simulink library "LIBRARY_SAD"  (R2025b)
settings: Solver=VariableStepAuto  StartTime=0.0  StopTime=10.0  RelTol=1e-3
values from neighbouring files (symbols this model uses):
  c = astroConstants(5)*1e3    [SCRIPT_SAD_DEMO.m]
  eps_E = deg2rad(astroConstants(63))    [SCRIPT_SAD_DEMO.m]
  F0 = 237    [SCRIPT_SAD_DEMO.m]
  F_e = 1358    [SCRIPT_SAD_DEMO.m]
  g = zeros(N, N+1)    [SCRIPT_SAD_DEMO.m]
  h = zeros(N, N+1)    [SCRIPT_SAD_DEMO.m]
  j_B = [0.01; 0.05; 0.01]    [SCRIPT_SAD_DEMO.m]
  JD0 = juliandate(startTime)    [SCRIPT_SAD_DEMO.m]
  mu = astroConstants(13)    [SCRIPT_SAD_DEMO.m]
  n = sqrt( (mu/ (a)^3))    [SCRIPT_SAD_DEMO.m]
  N = 13    [SCRIPT_SAD_DEMO.m]
  n_sun = 2*pi/T_sun    (= 1.99238499086e-07)    [SCRIPT_SAD_DEMO.m]
  r_sun = 1*AU    [SCRIPT_SAD_DEMO.m]
  Re = astroConstants(23)    [SCRIPT_SAD_DEMO.m]
  SRP = SRP_nom    [SCRIPT_SAD_DEMO.m]
  t0 = 0    [SCRIPT_SAD_DEMO.m]
  theta = 0    [SCRIPT_SAD_DEMO.m]
  w0 = w0_nom    [SCRIPT_SAD_DEMO.m]
  w_E = deg2rad(15.04)/3600    [SCRIPT_SAD_DEMO.m]
undefined symbols (not defined in the file or in its folder): g0_1, g1_1, h1_1, Ix, Iy, Iz, phi0, psi0, theta0
libraries: matrix_library x13, lIBRARY_SAD_SAD x12, $bdroot x5, LIBRARY_SAD_SAD x3, simulink x1
(part 2 of 2)

== system LIBRARY_SAD/Solar Radiation Torque (SRP)/Panel 3 ==
  Constant : Constant  Value=SRP.panel3.A
  Constant1 : Constant  Value=SRP.panel3.N_hat
  Constant2 : Constant  Value=SRP.panel3.rho_s
  Constant3 : Constant  Value=SRP.panel3.rho_d
  A_i : Outport
  N_B_hat_i : Outport  Port=2
  rho_s_i : Outport  Port=3
  rho_d_i : Outport  Port=4
  wires:
  Constant/1 -> A_i/1
  Constant1/1 -> N_B_hat_i/1
  Constant2/1 -> rho_s_i/1
  Constant3/1 -> rho_d_i/1

== system LIBRARY_SAD/Solar Radiation Torque (SRP)/Panel 4 ==
  Constant : Constant  Value=SRP.panel4.A
  Constant1 : Constant  Value=SRP.panel4.N_hat
  Constant2 : Constant  Value=SRP.panel4.rho_s
  Constant3 : Constant  Value=SRP.panel4.rho_d
  A_i : Outport
  N_B_hat_i : Outport  Port=2
  rho_s_i : Outport  Port=3
  rho_d_i : Outport  Port=4
  wires:
  Constant3/1 -> rho_d_i/1
  Constant2/1 -> rho_s_i/1
  Constant1/1 -> N_B_hat_i/1
  Constant/1 -> A_i/1

== system LIBRARY_SAD/Two-body Dynamics (keplerian elements)/Conic Equation ==
  a : Inport
  e : Inport  Port=2
  theta : Inport  Port=3
  Constant : Constant  Value=2
  Constant1 : Constant
  Constant2 : Constant
  Cos : Trigonometry  Operator=cos
  Divide : Product  Inputs=*/
  Power : Math  Operator=pow
  Product : Product
  Product1 : Product
  Sum : Sum  Inputs=+-
  Sum1 : Sum  Inputs=+-
  r : Outport
  wires:
  a/1 -> Product/1
  e/1 -> Product1/1, Power/1
  Constant/1 -> Power/2
  Power/1 -> Sum/2
  Constant1/1 -> Sum/1
  Sum/1 -> Product/2
  Product/1 -> Divide/1
  Divide/1 -> r/1
  Constant2/1 -> Sum1/1
  theta/1 -> Cos/1
  Cos/1 -> Product1/2
  Product1/1 -> Sum1/2
  Sum1/1 -> Divide/2

== system LIBRARY_SAD/Two-body Dynamics (keplerian elements)/Orbital Period ==
  a : Inport
  mu : Inport  Port=2
  Constant : Constant  Value=3
  Divide : Product  Inputs=*/
  Gain : Gain  Gain=2*pi
  Power : Math  Operator=pow
  Sqrt : Sqrt
  T : Outport
  wires:
  a/1 -> Power/1
  Constant/1 -> Power/2
  Power/1 -> Divide/1
  mu/1 -> Divide/2
  Divide/1 -> Sqrt/1
  Sqrt/1 -> Gain/1
  Gain/1 -> T/1

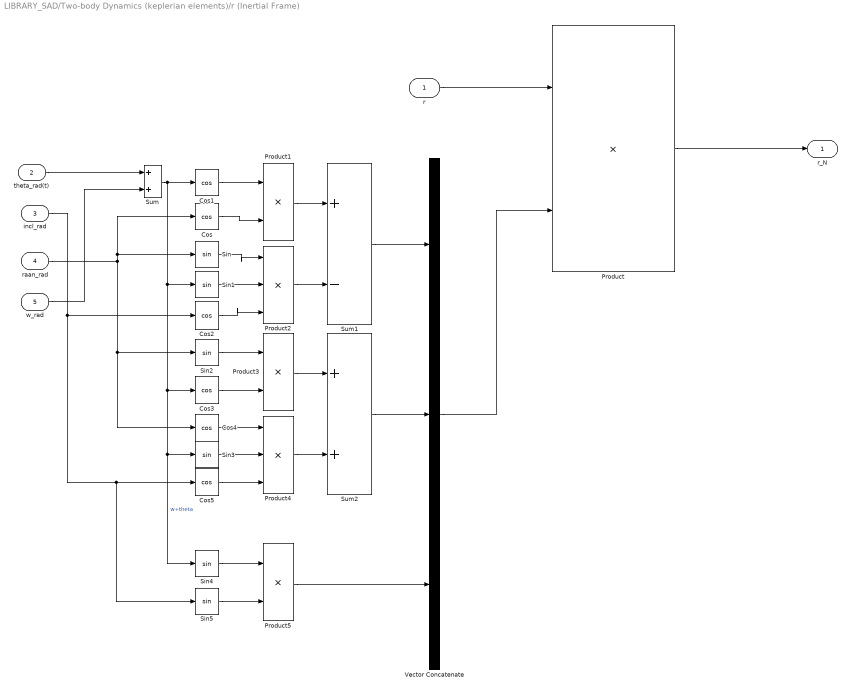
== system LIBRARY_SAD/Two-body Dynamics (keplerian elements)/r (Inertial Frame) ==
  r : Inport
  theta_rad(t) : Inport  Port=2
  incl_rad : Inport  Port=3
  raan_rad : Inport  Port=4
  w_rad : Inport  Port=5
  Cos{,1..5} (6 alike) : Trigonometry  Operator=cos
  Product{,1,3,5} (4 alike) : Product
  Product2 : Product  Inputs=3
  Product4 : Product  Inputs=3
  Sin{,1..5} (6 alike) : Trigonometry
  Sum : Sum
  Sum1 : Sum  Inputs=+-
  Sum2 : Sum
  Vector Concatenate : Concatenate  NumInputs=3
  r_N : Outport
  wires:
  r/1 -> Product/1
  raan_rad/1 -> Cos/1, Sin/1, Cos4/1, Sin2/1
  w_rad/1 -> Sum/2
  Cos/1 -> Product1/2
  theta_rad(t)/1 -> Sum/1
  Sum/1 -> Sin4/1, Sin3/1, Cos3/1, Sin1/1, Cos1/1  "w+theta"
  Cos1/1 -> Product1/1
  Product1/1 -> Sum1/1
  Product2/1 -> Sum1/2
  Sin/1 -> Product2/1
  Sin1/1 -> Product2/2
  Cos2/1 -> Product2/3
  incl_rad/1 -> Sin5/1, Cos5/1, Cos2/1
  Sum1/1 -> Vector Concatenate/1
  Sum2/1 -> Vector Concatenate/2
  Sin2/1 -> Product3/1
  Cos3/1 -> Product3/2
  Product3/1 -> Sum2/1
  Product4/1 -> Sum2/2
  Cos4/1 -> Product4/1
  Sin3/1 -> Product4/2
  Cos5/1 -> Product4/3
  Sin4/1 -> Product5/1
  Sin5/1 -> Product5/2
  Product5/1 -> Vector Concatenate/3
  Vector Concatenate/1 -> Product/2
  Product/1 -> r_N/1

== system LIBRARY_SAD/Magnetic Torque (Simple Dipole Model) /B_N (Simple Dipole Model)/Earth's Magnetic Dipole (unit vector) ==
  Time : Inport
  Constant : Constant  Value=11.5
  Constant1 : Constant  Value=11.5
  Constant2 : Constant  Value=11.5
  Cos : Trigonometry  Operator=cos
  Cos1 : Trigonometry
  Gain : Gain  Gain=w_E
  Gain1 : Gain  Gain=pi/180
  Gain2 : Gain  Gain=w_E
  Gain3 : Gain  Gain=pi/180
  Gain4 : Gain  Gain=pi/180
  Product : Product
  Product1 : Product
  Sin : Trigonometry
  Sin1 : Trigonometry
  Sin2 : Trigonometry  Operator=cos
  Vector Concatenate : Concatenate  NumInputs=3
  m_hat : Outport
  wires:
  Gain/1 -> Cos/1
  Cos/1 -> Product/1
  Sin/1 -> Product/2
  Constant/1 -> Gain1/1
  Gain1/1 -> Sin/1
  Product/1 -> Vector Concatenate/1
  Product1/1 -> Vector Concatenate/2
  Cos1/1 -> Product1/1
  Gain2/1 -> Cos1/1
  Time/1 -> Gain2/1, Gain/1
  Constant2/1 -> Gain4/1
  Gain4/1 -> Sin2/1
  Sin2/1 -> Vector Concatenate/3
  Vector Concatenate/1 -> m_hat/1  "m_hat"
  Gain3/1 -> Sin1/1
  Constant1/1 -> Gain3/1
  Sin1/1 -> Product1/2

== system LIBRARY_SAD/Magnetic Torque (Simple Dipole Model) /B_N (Simple Dipole Model)/H_0 ==
  Constant1 : Constant  Value=2
  Constant2 : Constant  Value=2
  Constant3 : Constant  Value=g0_1
  Constant4 : Constant  Value=g1_1
  Constant5 : Constant  Value=2
  Constant6 : Constant  Value=h1_1
  Power : Math  Operator=pow
  Power1 : Math  Operator=pow
  Power2 : Math  Operator=pow
  Sqrt : Sqrt
  Sum : Sum  Inputs=+++
  H_0 : Outport
  wires:
  Constant3/1 -> Power/1
  Power2/1 -> Sum/3
  Power1/1 -> Sum/2
  Sqrt/1 -> H_0/1
  Power/1 -> Sum/1
  Sum/1 -> Sqrt/1
  Constant1/1 -> Power/2
  Constant2/1 -> Power1/2
  Constant4/1 -> Power1/1
  Constant6/1 -> Power2/1
  Constant5/1 -> Power2/2

== matlab function LIBRARY_SAD/B_N (IGRF Model - Order N)/MATLAB Function1 ==
  data: alpha_G0 input; alpha_G output; w_E input; t0 input; t input
function alpha_G = alpha_G(alpha_G0,w_E,t0,t)
% ALPHA_G This function returns the Right ascension of Greenwich meridian
% in time, given a particular date (alpha_G0)
% INPUTS : alpha_G0 : Initial LST of Greenwhich [rad]
%           w_E : Average angular velocity of the Earth [rad/s]
%           t0 : Starting time [s]
%           t : Simulation time [s]
%
% OUTPUTS : alpha_G : Right Ascension of Greenwhich evolving with time [rad]

alpha_G = mod( alpha_G0 + w_E * (t - t0), 2*pi);

end

== matlab function LIBRARY_SAD/B_N (IGRF Model - Order N)/MATLAB Function2 ==
  data: r_SC_N input; alpha output; dec output
function [alpha,dec] = alpha_and_dec_from_r(r_SC_N)
%RA_AND_DEC_FROM_R This function computes the RA and declination (in Earth
%Equatorial Inertial Frame) given the vector r

% INPUTS: r : position vector  in EC/EQ

% OUTPUTS : ra: Right Ascension in Earth Centered Equatorial Inertial Frame
%               [rad]
%           dec: Declination in Earth Centred Equatorial Inertial frame [rad]

% Direction cosine
n = r_SC_N(3)/norm(r_SC_N);

% Computing declination
dec = asin(n);

% Computing right ascension
alpha = mod(atan2(r_SC_N(2),r_SC_N(1)), 2*pi);

end

== matlab function LIBRARY_SAD/B_N (IGRF Model - Order N)/MATLAB Function3 ==
  data: JD input; alpha_G0 output
function alpha_G0 = compute_alpha_G0(JD)
% COMPUTE_ALPHA_G0 This function computes Greenwich Sidereal Time at given Julian Date
% INPUTS: JD : Julian date [scalar]
% 
% OUTPUTS : Right ascension of Greenwich [rad]
D = JD - 2451545.0; % days since J2000.0
GST_deg = 280.46061837 + 360.98564736629 * D;
alpha_G0 = mod(GST_deg * pi/180, 2*pi); 
end

== matlab function LIBRARY_SAD/B_N (IGRF Model - Order N)/MATLAB Function4 ==
  data: r input; alpha_G input; B output; lon input; lat input; g input; h input; Re input; N input
function B = B_IGRF(r,alpha_G,lon,lat,g,h,Re,N)
% B_IGRF This function returns the magnetic field vector in the geocentric
% inertial frame (N)
% INPUTS: r:            norm of the position vector of the S/C in the inertial geocentric frame (N) [km]
%         alpha_G :     Right ascension of Greenwich [rad]
%         lon :         East longitude from Greenwich [rad]
%         lat :         Latitude, positive from equatorial plane (same as
%                       declination) [rad]
%         g :           IGRF 2025 'g' Gaussian coefficients, tabulated and
%                       taken from 'IGRF14coeffs.xlsx' [nT]
%         h :           IGRF 2025 'h' Gaussian coefficients, tabulated and
%                       taken from 'IGRF14coeffs.xlsx' [nT]
%         Re :          Equatorial radius of the Earth [km]
%         N :           Order of the IGRF Model Expansion
%
% OUTPUTS : B : Magnetic Field in the point (r,theta,phi), in ECI frame [T]

phi = lon;              % 'Azimuth' angle, same as longitude [rad]
theta = (pi/2-lat);     % Co-latitude, positive from z-axis of the ECEF Frame [rad]
alpha = phi + alpha_G;  % Right ascension of the S/C, in ECEF Frame

%% P-dP
% validated through the P and dP tables in "Jeremy Davis, Mathematical Modeling of Earth's Magnetic
% Field, 2004"

% P_{(n),(m+1)}: 
% given P(a,b) -> n=a, m=b-1
% n from 1 to N
% m from 0 to N
% N order of accuracy


% Initializing matrices. Rows: from 1 to N (n), Columns: from 0 to n (m)
K = zeros(N, N+1); 
P = zeros(N,N+1);
dP = zeros(N,N+1);

% Compute K coefficients for recursive formulas of P_{n,m}
for n = 1:N
    for m = 0:n
        if n == 1
            K(n, m+1) = 0;
        else
            K(n, m+1) = ((n-1)^2 - m^2) / ((2*n - 1)*(2*n - 3));
        end
    end
end


P_00 = 1;
dP_00 = 0;

P_01 = 0; 
dP_01 = 0;

P(1,1) = cos(theta); % n=1, m=0
dP(1,1) = -sin(theta)*P_00; 

P(1,2) = sin(theta);  % n=1, m=1
dP(1,2) = cos(theta)*P_00;

% Computation of Gaussian normalized associated Legendre Polynomials
for ii = 2:N % cycle for n from n=2 to n=N
    for jj = 0:ii % cycle fro m from m=0 to m=n
        if jj == ii
        P(ii,jj+1) = sin(theta)*P(ii-1,jj);
        dP(ii,jj+1) = sin(theta)*dP(ii-1,jj) + cos(theta)*P(ii-1,jj);
        elseif ii < 3
            if jj == 0 % n=2, m=0
            P(ii,jj+1) = cos(theta)*P(ii-1,jj+1) - K(ii,jj+1)*P_00;
            dP(ii,jj+1) = -sin(theta)*P(ii-1,jj+1) + cos(theta)*dP(ii-1,jj+1) ...
                        - K(ii,jj+1)*dP_00;
            elseif jj == 1 % n=2, m=1
                P(ii,jj+1) = cos(theta)*P(ii-1,jj+1) - K(ii,jj+1)*P_01;
                dP(ii,jj+1) = -sin(theta)*P(ii-1,jj+1) + cos(theta)*dP(ii-1,jj+1)...
                            - K(ii,jj+1)*dP_01;
            end
        else
            P(ii,jj+1) = cos(theta)*P(ii-1,jj+1) - K(ii,jj+1)*P(ii-2,jj+1);
            dP(ii,jj+1) = -sin(theta)*P(ii-1,jj+1) + cos(theta)*dP(ii-1,jj+1) ...
                        - K(ii,jj+1)*dP(ii-2,jj+1);
        end
    end
end

%% Magnetic Field

B_r = 0;
B_th = 0;
B_phi = 0;

for m = 0:N
    for n = 1:N
        if m<=n
            B_r = B_r + (Re/r)^(n+2)*(n+1)*...
                ((g(n,m+1)*cos(m*phi) + h(n,m+1)*sin(m*phi))*P(n, m+1));
            B_th = B_th + (Re/r)^(n+2)*...
                ((g(n,m+1)*cos(m*phi) + h(n,m+1)*sin(m*phi))*dP(n, m+1));
            B_phi = B_phi + (Re/r)^(n+2)*...
                (m*(-g(n,m+1)*sin(m*phi) + h(n,m+1)*cos(m*phi))* P(n, m+1));
        end
    end
end

B_th = -B_th;
B_phi = -B_phi/sin(theta);

B_x = ( B_r*cos(lat) + B_th*sin(lat) ) * cos(alpha) - B_phi*sin(alpha);
B_y = ( B_r*cos(lat) + B_th*sin(lat) ) * sin(alpha) + B_phi*cos(alpha);
B_z = B_r*sin(lat) - B_th*cos(lat);

B = [B_x*1e-9, B_y*1e-9, B_z*1e-9]'; %[T]
